simulink model "legacy_code_call_c_demo"  (R2021a)
settings: Solver=FixedStepDiscrete  StartTime=0.0  StopTime=10.0  RelTol=1e-3
PreLoadFcn:
  |  Simulink.importExternalCTypes('./C_Files/ex_myTypes_LCT.h');
  | structParam = struct;
  | structParam.param1 = 15;
  | structParam.param2 = 20;
  | structParam.param3 = 5;
CloseFcn:
  | try
  | rmdir slprj\ s
  | catch
  | end
  | try
  | folder_name = [bdroot '*'];
  | rmdir(folder_name,'s')
  | catch
  | end
  | try
  | file_temp_name = [bdroot '.slxc'];
  | delete(file_temp_name)
  | catch
  | end
  | clear folder_name file_temp_name
settings Model: Creator=jetson  LastModifiedBy=jetson
settings DataIOCC: SaveOutput=off  SignalLogging=off  DSMLogging=off  SaveTime=off  ReturnWorkspaceOutputs=off
settings OptimizationCC: DefaultParameterBehavior=Inlined  EnhancedBackFolding=on  PassReuseOutputArgsAs=Individual arguments  ZeroExternalMemoryAtStartup=off  ZeroInternalMemoryAtStartup=off  OptimizeBlockOrder=speed  DifferentSizesBufferReuse=on  OptimizationCustomize=off  EfficientTunableParamExpr=on
settings DebuggingCC: ParameterTunabilityLossMsg=error
settings SFSimCC: MATLABDynamicMemAlloc=off
settings RTWCC: SystemTargetFile=ert.tlc  GenCodeOnly=on  TemplateMakefile=ert_default_tmf  GenerateReport=on  IncludeHyperlinkInReport=on  LaunchReport=on  GenerateTraceInfo=on
settings CodeAppCC: ForceParamTrailComments=on  IgnoreCustomStorageClasses=off  OperatorAnnotations=on  SimulinkDataObjDesc=on  SFDataObjDesc=on  InsertBlockDesc=on
settings ERTTargetCC: TargetLangStandard=C99 (ISO)  GenerateSampleERTMain=on  InlinedParameterPlacement=NonHierarchical  ERTCustomFileTemplate=example_file_process.tlc

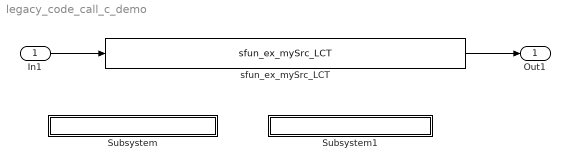
== system legacy_code_call_c_demo ==
  In1 : Inport  OutDataTypeStr=Bus: sigStructType
      settings: AttributesFormatString=%<OutDataTypeStr>
  Subsystem : Subsystem
      settings: OpenFcn=web(fullfile(docroot, 'simulink/sfg/integrating-existing-c-functions-into-simulink-models-with-the-legacy-code-tool.html'))
      mask Display: disp('double click open help')
  Subsystem1 : Subsystem
      settings: OpenFcn=edit legacy_code_demo.m
      mask Display: disp('double click open script')
  sfun_ex_mySrc_LCT : S-Function  FunctionName=sfun_ex_mySrc_LCT  Parameters=SParameter1  SFunctionDeploymentMode=off  EnableBusSupport=off  mask(Legacy Function){SFunctionSpec=void myFcn(sigStructType u1[1], paramStructType p1[1], sigStructType y1[1]), SParameter1=structParam, ShowSpec=on}
      mask prompts: SParameter1 "P1:"; ShowSpec "Display function specification"
      mask help:
      | This block allows you to call the legacy functions specified by the following Legacy Code Tool definition:
      | def.SFunctionName = 'sfun_ex_mySrc_LCT';
      | def.OutputFcnSpec = 'void myFcn(sigStructType u1[1], paramStructType p1[1], sigStructType y1[1])';
      | def.HeaderFiles = {'ex_myTypes_LCT.h'};
      mask Help: <p>This block was generated automatically by the Legacy Code Tool. For detailed help on this tool, call<a href="matlab:legacy_code('help')"> legacy_code('help')</a>.</p>
      mask Callback ShowSpec:
      | if strcmp(get_param(gcbh, 'ShowSpec'), 'on')
      |   set_param(gcbh, 'MaskDisplay', sprintf('fprintf(''%s'');', get_param(gcbh, 'SFunctionSpec')));
      | else
      |   set_param(gcbh, 'MaskDisplay', sprintf('fprintf(''%s'');', get_param(gcbh, 'FunctionName')));
      | end
      mask Display: fprintf('void myFcn(sigStructType u1[1], paramStructType p1[1], sigStructType y1[1])');
  Out1 : Outport  OutDataTypeStr=Bus: sigStructType
      settings: AttributesFormatString=%<OutDataTypeStr>
  wires:
  In1/1 -> sfun_ex_mySrc_LCT/1
  sfun_ex_mySrc_LCT/1 -> Out1/1

== system legacy_code_call_c_demo/Subsystem ==

== system legacy_code_call_c_demo/Subsystem1 ==
